simulink model "two_time_domains"  (R2025b)
settings: Solver=ode23tb  StartTime=0.0  StopTime=simlength  MaxStep=tc
undefined symbols (not defined in the file): dead_time_AFE, enable_pwm_phase_corrections, ki_align, kp_align, lim_down_align, lim_up_align, omega_base, tc, time_gain_afe_module_1, time_gain_afe_module_2, time_gain_inv_module_1, time_gain_inv_module_2, tPWM_AFE, tPWM_INV, ts_afe, ts_inv
settings Model: Creator=dbagn  LastModifiedBy=dbagn
settings SolverCC: NumberNewtonIterations=3.0  ZeroCrossControl=DisableAll  AlgebraicLoopSolver=TrustRegion  SolverResetMethod=Robust  AutoInsertRateTranBlk=on
settings DataIOCC: SaveOutput=off  SignalLogging=off  DSMLogging=off  SaveTime=off  ReturnWorkspaceOutputs=off
settings OptimizationCC: ReuseModelBlockBuffer=off
settings DebuggingCC: UnconnectedInputMsg=warning  UnconnectedOutputMsg=warning  UnconnectedLineMsg=warning
settings ModelReferenceCC: UpdateModelReferenceTargets=Force  EnableRefExpFcnMdlSchedulingChecks=on  ParallelModelReferenceMATLABWorkerInit=Copy Base Workspace
settings SFSimCC: CustomCodeUndefinedFunction=ThrowError  DefaultCustomCodeDeterministicFunctions=All
settings RTWCC: GPUComputeCapability=3.5  DLArmComputeVersion=19.05

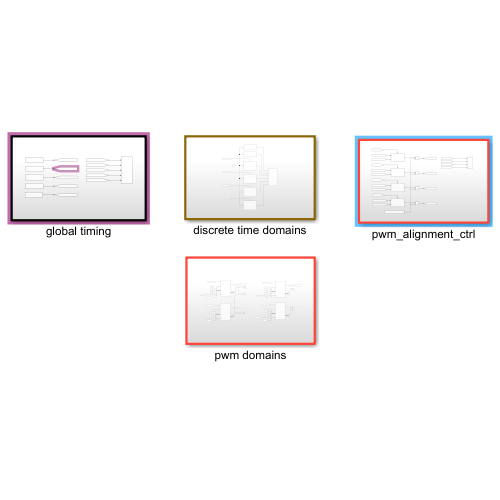
[thumbnail: Simulink's stored preview of the top-level diagram]
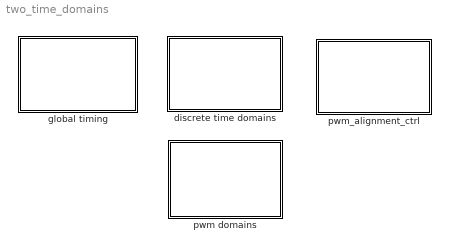
== system two_time_domains ==
  discrete time domains : Subsystem
  global timing : Subsystem
  pwm domains : Subsystem
  pwm_alignment_ctrl : Subsystem

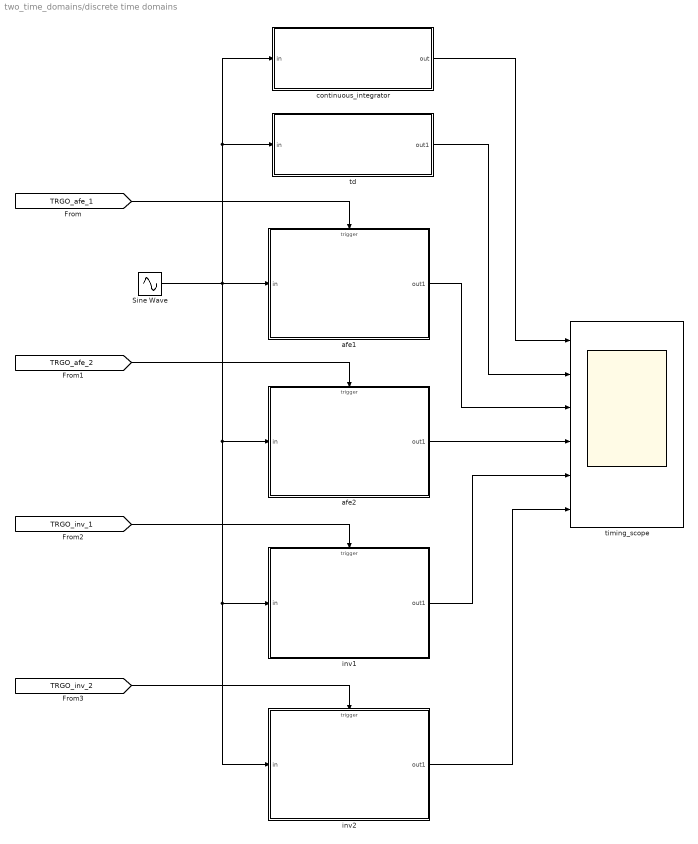
== system two_time_domains/discrete time domains ==
  Sine Wave : Sin  Frequency=omega_base  SampleTime=0
  afe1 : Subsystem
  afe2 : Subsystem
  continuous_integrator : Subsystem
  inv1 : Subsystem
  inv2 : Subsystem
  td : Subsystem
  timing_scope : Scope  NumInputPorts=6
      settings: SampleTime=tc  ActiveDisplayYMinimum=-0.89002047717580246  ActiveDisplayYMaximum=0.93911648822902838
  wires:
  [TRGO_afe_1] -> afe1/Trigger
  [TRGO_afe_2] -> afe2/Trigger
  Sine Wave/1 -> td/1(in), continuous_integrator/1(in), afe1/1(in), inv2/1(in), inv1/1(in), afe2/1(in)
  [TRGO_inv_2] -> inv2/Trigger
  [TRGO_inv_1] -> inv1/Trigger
  afe1/1(out1) -> timing_scope/3
  afe2/1(out1) -> timing_scope/4
  inv1/1(out1) -> timing_scope/5
  inv2/1(out1) -> timing_scope/6
  td/1(out1) -> timing_scope/2
  continuous_integrator/1(out) -> timing_scope/1

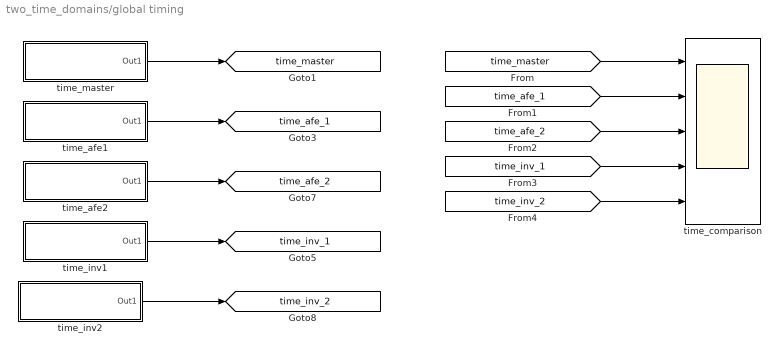
== system two_time_domains/global timing ==
  time_afe1 : Subsystem  mask{k=time_gain_afe_module_1}
      mask prompts: k "Time Gain"
      mask Display:
      | disp('time-gen');
      | port_label('output', 1, 'tout');
  time_afe2 : Subsystem  mask{k=time_gain_afe_module_2}
      mask prompts: k "Time Gain"
      mask Display:
      | disp('time-gen');
      | port_label('output', 1, 'tout');
  time_comparison : Scope  NumInputPorts=5
      settings: ActiveDisplayYMinimum=-0.0261093772199036  ActiveDisplayYMaximum=0.23498439497913245  DataLoggingVariableName=ScopeData6
  time_inv1 : Subsystem  mask{k=time_gain_inv_module_1}
      mask prompts: k "Time Gain"
      mask Display:
      | disp('time-gen');
      | port_label('output', 1, 'tout');
  time_inv2 : Subsystem  mask{k=time_gain_inv_module_2}
      mask prompts: k "Time Gain"
      mask Display:
      | disp('time-gen');
      | port_label('output', 1, 'tout');
  time_master : Subsystem  mask{k=1}
      mask prompts: k "Time Gain"
      mask Display:
      | disp('master');
      | port_label('output', 1, 'time');
  tag scope: time_afe_1=global, time_afe_2=global, time_inv_1=global, time_inv_2=global, time_master=global
  wires:
  time_afe1/1(Out1) -> [time_afe_1]
  time_afe2/1(Out1) -> [time_afe_2]
  time_master/1(Out1) -> [time_master]
  time_inv2/1(Out1) -> [time_inv_2]
  time_inv1/1(Out1) -> [time_inv_1]
  [time_master] -> time_comparison/1
  [time_afe_1] -> time_comparison/2
  [time_afe_2] -> time_comparison/3
  [time_inv_1] -> time_comparison/4
  [time_inv_2] -> time_comparison/5

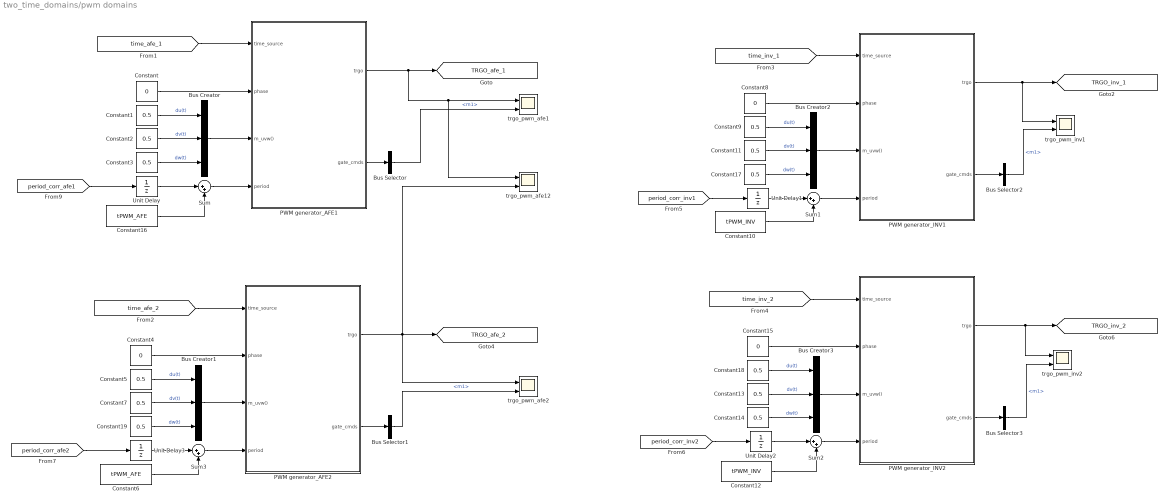
== system two_time_domains/pwm domains ==
  Bus Creator{,1..3} (4 alike) : BusCreator  Inputs=3
  Bus Selector{,1..3} (4 alike) : BusSelector  OutputSignals=m1
  Constant{,4,8,15} (4 alike) : Constant  Value=0
  Constant{1..3,5,7,9,11,13..14,17..19} (12 alike) : Constant  Value=0.5
  Constant10 : Constant  Value=tPWM_INV
  Constant12 : Constant  Value=tPWM_INV
  Constant16 : Constant  Value=tPWM_AFE
  Constant6 : Constant  Value=tPWM_AFE
  PWM generator_AFE1 : Subsystem  mask{m_up=0.98, m_low=0.02, dead_time=dead_time_AFE, pos_cmd_gate=15, neg_cmd_gate=-10, polarity=1, tc=tc}
      mask prompts: m_up "Max Input Modulation Value"; m_low "Min Input Modulation Value"; dead_time "Dead Time (s)"; pos_cmd_gate "Positive Gate Voltage (V)"; neg_cmd_gate "Negative Gate Voltage (V)"; polarity "Polarity (pu)"; tc "Sampling time"
  PWM generator_AFE2 : Subsystem  mask{m_up=0.98, m_low=0.02, dead_time=dead_time_AFE, pos_cmd_gate=15, neg_cmd_gate=-10, polarity=1, tc=tc}
      mask prompts: m_up "Max Input Modulation Value"; m_low "Min Input Modulation Value"; dead_time "Dead Time (s)"; pos_cmd_gate "Positive Gate Voltage (V)"; neg_cmd_gate "Negative Gate Voltage (V)"; polarity "Polarity (pu)"; tc "Sampling time"
  PWM generator_INV1 : Subsystem  mask{m_up=0.98, m_low=0.02, dead_time=dead_time_AFE, pos_cmd_gate=15, neg_cmd_gate=-10, polarity=1, tc=tc}
      mask prompts: m_up "Max Input Modulation Value"; m_low "Min Input Modulation Value"; dead_time "Dead Time (s)"; pos_cmd_gate "Positive Gate Voltage (V)"; neg_cmd_gate "Negative Gate Voltage (V)"; polarity "Polarity (pu)"; tc "Sampling time"
  PWM generator_INV2 : Subsystem  mask{m_up=0.98, m_low=0.02, dead_time=dead_time_AFE, pos_cmd_gate=15, neg_cmd_gate=-10, polarity=1, tc=tc}
      mask prompts: m_up "Max Input Modulation Value"; m_low "Min Input Modulation Value"; dead_time "Dead Time (s)"; pos_cmd_gate "Positive Gate Voltage (V)"; neg_cmd_gate "Negative Gate Voltage (V)"; polarity "Polarity (pu)"; tc "Sampling time"
  Sum{,1..3} (4 alike) : Sum  Inputs=|++
  Unit Delay{,1..3} (4 alike) : UnitDelay  InitialCondition=1  SampleTime=tc  HasFrameUpgradeWarning=on
  trgo_pwm_afe1 : Scope  NumInputPorts=2
      settings: ActiveDisplayYMinimum=-11.375  ActiveDisplayYMaximum=2.375
  trgo_pwm_afe12 : Scope  NumInputPorts=2
      settings: ActiveDisplayYMinimum=-1  ActiveDisplayYMaximum=1  DataLoggingVariableName=ScopeData5
  trgo_pwm_afe2 : Scope  NumInputPorts=2
      settings: ActiveDisplayYMinimum=-0.12499999999999997  ActiveDisplayYMaximum=1.125  DataLoggingVariableName=ScopeData2
  trgo_pwm_inv1 : Scope  NumInputPorts=2
      settings: ActiveDisplayYMinimum=-0.12499999999999997  ActiveDisplayYMaximum=1.125  DataLoggingVariableName=ScopeData3
  trgo_pwm_inv2 : Scope  NumInputPorts=2
      settings: ActiveDisplayYMinimum=-0.12499999999999997  ActiveDisplayYMaximum=1.125  DataLoggingVariableName=ScopeData4
  tag scope: TRGO_afe_1=global, TRGO_afe_2=global, TRGO_inv_1=global, TRGO_inv_2=global
  wires:
  Constant/1 -> PWM generator_AFE1/2(phase)
  Constant1/1 -> Bus Creator/1  "du(t)"
  [time_afe_1] -> PWM generator_AFE1/1(time_source)
  Bus Creator/1 -> PWM generator_AFE1/3(m_uvw())
  PWM generator_AFE1/1(trgo) -> trgo_pwm_afe12/1, trgo_pwm_afe1/1, [TRGO_afe_1]
  Constant2/1 -> Bus Creator/2  "dv(t)"
  Constant3/1 -> Bus Creator/3  "dw(t)"
  PWM generator_AFE1/2(gate_cmds) -> Bus Selector/1
  Bus Selector/1 -> trgo_pwm_afe1/2  "<m1>"
  Bus Selector1/1 -> trgo_pwm_afe2/2  "<m1>"
  PWM generator_AFE2/2(gate_cmds) -> Bus Selector1/1
  PWM generator_AFE2/1(trgo) -> trgo_pwm_afe12/2, [TRGO_afe_2], trgo_pwm_afe2/1
  [time_afe_2] -> PWM generator_AFE2/1(time_source)
  [time_inv_2] -> PWM generator_INV2/1(time_source)
  PWM generator_INV2/1(trgo) -> trgo_pwm_inv2/1, [TRGO_inv_2]
  PWM generator_INV2/2(gate_cmds) -> Bus Selector3/1
  Bus Selector3/1 -> trgo_pwm_inv2/2  "<m1>"
  Bus Selector2/1 -> trgo_pwm_inv1/2  "<m1>"
  PWM generator_INV1/2(gate_cmds) -> Bus Selector2/1
  PWM generator_INV1/1(trgo) -> [TRGO_inv_1], trgo_pwm_inv1/1
  [time_inv_1] -> PWM generator_INV1/1(time_source)
  Unit Delay/1 -> Sum/1
  [period_corr_afe1] -> Unit Delay/1
  Constant16/1 -> Sum/2
  Sum/1 -> PWM generator_AFE1/4(period)
  Constant10/1 -> Sum1/2
  [period_corr_inv1] -> Unit Delay1/1
  Constant9/1 -> Bus Creator2/1  "du(t)"
  Constant8/1 -> PWM generator_INV1/2(phase)
  Constant17/1 -> Bus Creator2/3  "dw(t)"
  Unit Delay1/1 -> Sum1/1
  Bus Creator2/1 -> PWM generator_INV1/3(m_uvw())
  Constant11/1 -> Bus Creator2/2  "dv(t)"
  Constant13/1 -> Bus Creator3/2  "dv(t)"
  Bus Creator3/1 -> PWM generator_INV2/3(m_uvw())
  Unit Delay2/1 -> Sum2/1
  Constant14/1 -> Bus Creator3/3  "dw(t)"
  Constant15/1 -> PWM generator_INV2/2(phase)
  Constant18/1 -> Bus Creator3/1  "du(t)"
  [period_corr_inv2] -> Unit Delay2/1
  Sum2/1 -> PWM generator_INV2/4(period)
  Constant12/1 -> Sum2/2
  Constant6/1 -> Sum3/2
  Sum3/1 -> PWM generator_AFE2/4(period)
  [period_corr_afe2] -> Unit Delay3/1
  Constant5/1 -> Bus Creator1/1  "du(t)"
  Constant4/1 -> PWM generator_AFE2/2(phase)
  Constant19/1 -> Bus Creator1/3  "dw(t)"
  Unit Delay3/1 -> Sum3/1
  Bus Creator1/1 -> PWM generator_AFE2/3(m_uvw())
  Constant7/1 -> Bus Creator1/2  "dv(t)"
  Sum1/1 -> PWM generator_INV1/4(period)

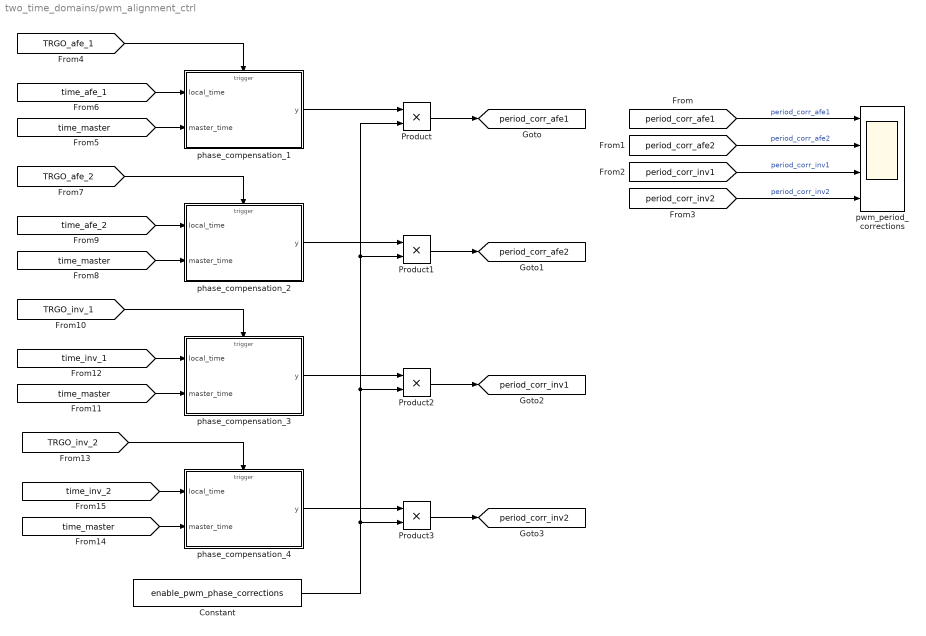
== system two_time_domains/pwm_alignment_ctrl ==
  Constant : Constant  Value=enable_pwm_phase_corrections
  Product{,1..3} (4 alike) : Product
  phase_compensation_1 : Subsystem
  phase_compensation_2 : Subsystem
  phase_compensation_3 : Subsystem
  phase_compensation_4 : Subsystem
  pwm_period_corrections : Scope  NumInputPorts=4
      settings: ActiveDisplayString=4  ActiveDisplayYMinimum=-6.4875940874999986E-5  ActiveDisplayYMaximum=7.2084378749999972E-6  DataLoggingVariableName=ScopeData7
  tag scope: period_corr_afe1=global, period_corr_afe2=global, period_corr_inv1=global, period_corr_inv2=global
  wires:
  Constant/1 -> Product1/2, Product/2, Product2/2, Product3/2
  Product/1 -> [period_corr_afe1]
  Product1/1 -> [period_corr_afe2]
  Product2/1 -> [period_corr_inv1]
  Product3/1 -> [period_corr_inv2]
  [period_corr_afe1] -> pwm_period_corrections/1  "period_corr_afe1"
  [period_corr_afe2] -> pwm_period_corrections/2  "period_corr_afe2"
  [period_corr_inv1] -> pwm_period_corrections/3  "period_corr_inv1"
  [period_corr_inv2] -> pwm_period_corrections/4  "period_corr_inv2"
  phase_compensation_1/1(y) -> Product/1
  [time_afe_1] -> phase_compensation_1/1(local_time)
  [time_master] -> phase_compensation_1/2(master_time)
  [time_master] -> phase_compensation_2/2(master_time)
  [time_afe_2] -> phase_compensation_2/1(local_time)
  phase_compensation_2/1(y) -> Product1/1
  [time_inv_1] -> phase_compensation_3/1(local_time)
  [time_master] -> phase_compensation_3/2(master_time)
  phase_compensation_3/1(y) -> Product2/1
  [time_master] -> phase_compensation_4/2(master_time)
  [time_inv_2] -> phase_compensation_4/1(local_time)
  phase_compensation_4/1(y) -> Product3/1
  [TRGO_afe_1] -> phase_compensation_1/Trigger
  [TRGO_inv_2] -> phase_compensation_4/Trigger
  [TRGO_inv_1] -> phase_compensation_3/Trigger
  [TRGO_afe_2] -> phase_compensation_2/Trigger

== system two_time_domains/discrete time domains/afe1 ==
  in : Inport
  Trigger : TriggerPort  VariantControl=(inherit)  PortDimensions=1
  LPF1_1 : Subsystem  mask{ts=ts_afe, omega=omega_base}
      mask Display:
      | disp('LPF1');
      | port_label('input', 1, 'u');
      | port_label('output', 1, 'y');
  out1 : Outport
  wires:
  in/1 -> LPF1_1/1(u)
  LPF1_1/1(y) -> out1/1

== system two_time_domains/discrete time domains/afe2 ==
  in : Inport
  Trigger : TriggerPort  VariantControl=(inherit)  PortDimensions=1
  LPF1_1 : Subsystem  mask{ts=ts_afe, omega=omega_base}
      mask Display:
      | disp('LPF1');
      | port_label('input', 1, 'u');
      | port_label('output', 1, 'y');
  out1 : Outport
  wires:
  LPF1_1/1(y) -> out1/1
  in/1 -> LPF1_1/1(u)

== system two_time_domains/discrete time domains/continuous_integrator ==
  in : Inport
  Transfer Fcn : TransferFcn  Denominator=[1/omega_base 1]
  out : Outport
  wires:
  in/1 -> Transfer Fcn/1
  Transfer Fcn/1 -> out/1

== system two_time_domains/discrete time domains/inv1 ==
  in : Inport
  Trigger : TriggerPort  VariantControl=(inherit)  PortDimensions=1
  LPF1_1 : Subsystem  mask{ts=ts_inv, omega=omega_base}
      mask Display:
      | disp('LPF1');
      | port_label('input', 1, 'u');
      | port_label('output', 1, 'y');
  out1 : Outport
  wires:
  in/1 -> LPF1_1/1(u)
  LPF1_1/1(y) -> out1/1

== system two_time_domains/discrete time domains/inv2 ==
  in : Inport
  Trigger : TriggerPort  VariantControl=(inherit)  PortDimensions=1
  LPF1_1 : Subsystem  mask{ts=ts_inv, omega=omega_base}
      mask Display:
      | disp('LPF1');
      | port_label('input', 1, 'u');
      | port_label('output', 1, 'y');
  out1 : Outport
  wires:
  LPF1_1/1(y) -> out1/1
  in/1 -> LPF1_1/1(u)

== system two_time_domains/discrete time domains/td ==
  in : Inport
  LPF1_1 : Subsystem  mask{ts=tc, omega=omega_base}
      mask Display:
      | disp('LPF1');
      | port_label('input', 1, 'u');
      | port_label('output', 1, 'y');
  out1 : Outport
  wires:
  LPF1_1/1(y) -> out1/1
  in/1 -> LPF1_1/1(u)

== system two_time_domains/global timing/time_afe1 ==
  Gain : Gain  Gain=k
  time_1 : Clock
  Out1 : Outport
  wires:
  time_1/1 -> Gain/1
  Gain/1 -> Out1/1

== system two_time_domains/global timing/time_afe2 ==
  Gain : Gain  Gain=k
  time_1 : Clock
  Out1 : Outport
  wires:
  Gain/1 -> Out1/1
  time_1/1 -> Gain/1

== system two_time_domains/global timing/time_inv1 ==
  Gain : Gain  Gain=k
  time_1 : Clock
  Out1 : Outport
  wires:
  time_1/1 -> Gain/1
  Gain/1 -> Out1/1

== system two_time_domains/global timing/time_inv2 ==
  Gain : Gain  Gain=k
  time_1 : Clock
  Out1 : Outport
  wires:
  Gain/1 -> Out1/1
  time_1/1 -> Gain/1

== system two_time_domains/global timing/time_master ==
  Gain : Gain  Gain=k
  time_1 : Clock
  Out1 : Outport
  wires:
  Gain/1 -> Out1/1
  time_1/1 -> Gain/1

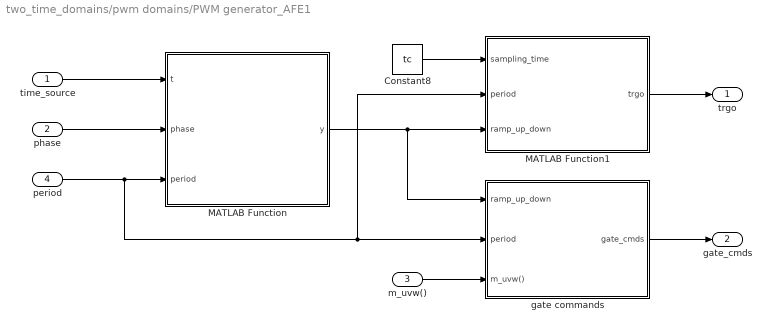
== system two_time_domains/pwm domains/PWM generator_AFE1 ==
  time_source : Inport
  phase : Inport  Port=2
  m_uvw() : Inport  Port=3
  period : Inport  Port=4
  Constant8 : Constant  Value=tc
  MATLAB Function : MATLAB Function  TreatAsAtomicUnit=on  SystemSampleTime=tc
  MATLAB Function1 : MATLAB Function  TreatAsAtomicUnit=on  SystemSampleTime=tc
  gate commands : Subsystem
  trgo : Outport
  gate_cmds : Outport  Port=2
  wires:
  phase/1 -> MATLAB Function/2(phase)
  MATLAB Function/1(y) -> gate commands/1(ramp_up_down), MATLAB Function1/3(ramp_up_down)
  MATLAB Function1/1(trgo) -> trgo/1
  Constant8/1 -> MATLAB Function1/1(sampling_time)
  period/1 -> MATLAB Function/3(period), MATLAB Function1/2(period), gate commands/2(period)
  m_uvw()/1 -> gate commands/3(m_uvw())
  gate commands/1(gate_cmds) -> gate_cmds/1
  time_source/1 -> MATLAB Function/1(t)

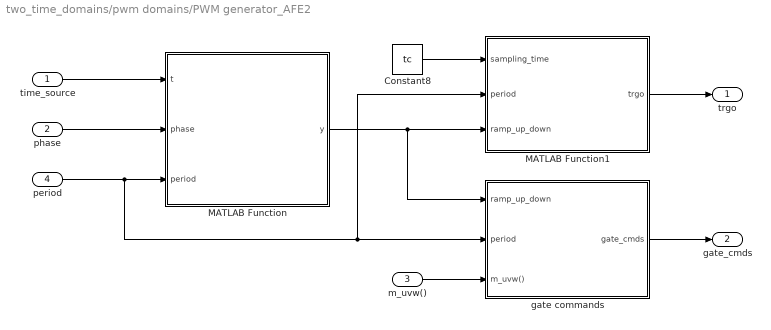
== system two_time_domains/pwm domains/PWM generator_AFE2 ==
  time_source : Inport
  phase : Inport  Port=2
  m_uvw() : Inport  Port=3
  period : Inport  Port=4
  Constant8 : Constant  Value=tc
  MATLAB Function : MATLAB Function  TreatAsAtomicUnit=on  SystemSampleTime=tc
  MATLAB Function1 : MATLAB Function  TreatAsAtomicUnit=on  SystemSampleTime=tc
  gate commands : Subsystem
  trgo : Outport
  gate_cmds : Outport  Port=2
  wires:
  time_source/1 -> MATLAB Function/1(t)
  gate commands/1(gate_cmds) -> gate_cmds/1
  m_uvw()/1 -> gate commands/3(m_uvw())
  period/1 -> gate commands/2(period), MATLAB Function1/2(period), MATLAB Function/3(period)
  Constant8/1 -> MATLAB Function1/1(sampling_time)
  MATLAB Function1/1(trgo) -> trgo/1
  MATLAB Function/1(y) -> MATLAB Function1/3(ramp_up_down), gate commands/1(ramp_up_down)
  phase/1 -> MATLAB Function/2(phase)

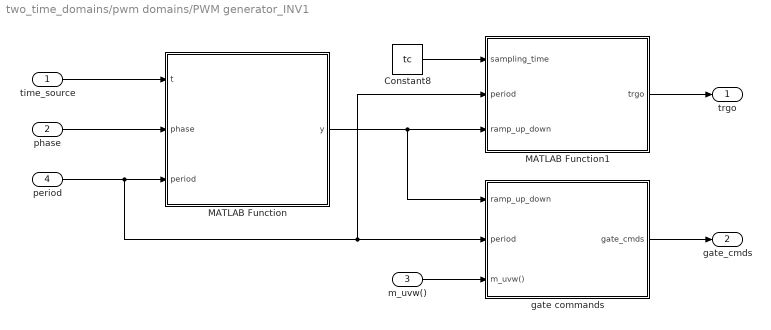
== system two_time_domains/pwm domains/PWM generator_INV1 ==
  time_source : Inport
  phase : Inport  Port=2
  m_uvw() : Inport  Port=3
  period : Inport  Port=4
  Constant8 : Constant  Value=tc
  MATLAB Function : MATLAB Function  TreatAsAtomicUnit=on  SystemSampleTime=tc
  MATLAB Function1 : MATLAB Function  TreatAsAtomicUnit=on  SystemSampleTime=tc
  gate commands : Subsystem
  trgo : Outport
  gate_cmds : Outport  Port=2
  wires:
  phase/1 -> MATLAB Function/2(phase)
  MATLAB Function/1(y) -> gate commands/1(ramp_up_down), MATLAB Function1/3(ramp_up_down)
  MATLAB Function1/1(trgo) -> trgo/1
  Constant8/1 -> MATLAB Function1/1(sampling_time)
  period/1 -> MATLAB Function/3(period), MATLAB Function1/2(period), gate commands/2(period)
  m_uvw()/1 -> gate commands/3(m_uvw())
  gate commands/1(gate_cmds) -> gate_cmds/1
  time_source/1 -> MATLAB Function/1(t)

== system two_time_domains/pwm domains/PWM generator_INV2 ==
  time_source : Inport
  phase : Inport  Port=2
  m_uvw() : Inport  Port=3
  period : Inport  Port=4
  Constant8 : Constant  Value=tc
  MATLAB Function : MATLAB Function  TreatAsAtomicUnit=on  SystemSampleTime=tc
  MATLAB Function1 : MATLAB Function  TreatAsAtomicUnit=on  SystemSampleTime=tc
  gate commands : Subsystem
  trgo : Outport
  gate_cmds : Outport  Port=2
  wires:
  time_source/1 -> MATLAB Function/1(t)
  gate commands/1(gate_cmds) -> gate_cmds/1
  m_uvw()/1 -> gate commands/3(m_uvw())
  period/1 -> gate commands/2(period), MATLAB Function1/2(period), MATLAB Function/3(period)
  Constant8/1 -> MATLAB Function1/1(sampling_time)
  MATLAB Function1/1(trgo) -> trgo/1
  MATLAB Function/1(y) -> MATLAB Function1/3(ramp_up_down), gate commands/1(ramp_up_down)
  phase/1 -> MATLAB Function/2(phase)

== system two_time_domains/pwm_alignment_ctrl/phase_compensation_1 ==
  local_time : Inport
  master_time : Inport  Port=2
  Trigger : TriggerPort  VariantControl=(inherit)  PortDimensions=1
  Gain1 : Gain  Gain=tPWM_AFE
  alignment_pictrl : Subsystem
  y : Outport
  wires:
  local_time/1 -> alignment_pictrl/1(local_time)
  master_time/1 -> alignment_pictrl/2(master_time)
  alignment_pictrl/1(dp) -> Gain1/1
  Gain1/1 -> y/1

== system two_time_domains/pwm_alignment_ctrl/phase_compensation_2 ==
  local_time : Inport
  master_time : Inport  Port=2
  Trigger : TriggerPort  VariantControl=(inherit)  PortDimensions=1
  Gain1 : Gain  Gain=tPWM_AFE
  alignment_pictrl : Subsystem
  y : Outport
  wires:
  alignment_pictrl/1(dp) -> Gain1/1
  master_time/1 -> alignment_pictrl/2(master_time)
  local_time/1 -> alignment_pictrl/1(local_time)
  Gain1/1 -> y/1

== system two_time_domains/pwm_alignment_ctrl/phase_compensation_3 ==
  local_time : Inport
  master_time : Inport  Port=2
  Trigger : TriggerPort  VariantControl=(inherit)  PortDimensions=1
  Gain1 : Gain  Gain=tPWM_INV
  alignment_pictrl : Subsystem
  y : Outport
  wires:
  local_time/1 -> alignment_pictrl/1(local_time)
  master_time/1 -> alignment_pictrl/2(master_time)
  alignment_pictrl/1(dp) -> Gain1/1
  Gain1/1 -> y/1

== system two_time_domains/pwm_alignment_ctrl/phase_compensation_4 ==
  local_time : Inport
  master_time : Inport  Port=2
  Trigger : TriggerPort  VariantControl=(inherit)  PortDimensions=1
  Gain1 : Gain  Gain=tPWM_INV
  alignment_pictrl : Subsystem
  y : Outport
  wires:
  alignment_pictrl/1(dp) -> Gain1/1
  master_time/1 -> alignment_pictrl/2(master_time)
  local_time/1 -> alignment_pictrl/1(local_time)
  Gain1/1 -> y/1

== system two_time_domains/discrete time domains/afe1/LPF1_1 ==
  u : Inport
  Gain : Gain  Gain=1-exp(-omega*ts)
  Gain1 : Gain  Gain=exp(-omega*ts)
  Sum : Sum  Inputs=|++
  Unit Delay : UnitDelay  SampleTime=-1  HasFrameUpgradeWarning=on
  y : Outport
  wires:
  Gain1/1 -> Sum/2
  Unit Delay/1 -> y/1, Gain1/1
  Gain/1 -> Sum/1
  Sum/1 -> Unit Delay/1
  u/1 -> Gain/1

== system two_time_domains/discrete time domains/afe2/LPF1_1 ==
  u : Inport
  Gain : Gain  Gain=1-exp(-omega*ts)
  Gain1 : Gain  Gain=exp(-omega*ts)
  Sum : Sum  Inputs=|++
  Unit Delay : UnitDelay  SampleTime=-1  HasFrameUpgradeWarning=on
  y : Outport
  wires:
  u/1 -> Gain/1
  Sum/1 -> Unit Delay/1
  Gain/1 -> Sum/1
  Unit Delay/1 -> Gain1/1, y/1
  Gain1/1 -> Sum/2

== system two_time_domains/discrete time domains/inv1/LPF1_1 ==
  u : Inport
  Gain : Gain  Gain=1-exp(-omega*ts)
  Gain1 : Gain  Gain=exp(-omega*ts)
  Sum : Sum  Inputs=|++
  Unit Delay : UnitDelay  SampleTime=-1  HasFrameUpgradeWarning=on
  y : Outport
  wires:
  Gain1/1 -> Sum/2
  Unit Delay/1 -> y/1, Gain1/1
  Gain/1 -> Sum/1
  Sum/1 -> Unit Delay/1
  u/1 -> Gain/1

== system two_time_domains/discrete time domains/inv2/LPF1_1 ==
  u : Inport
  Gain : Gain  Gain=1-exp(-omega*ts)
  Gain1 : Gain  Gain=exp(-omega*ts)
  Sum : Sum  Inputs=|++
  Unit Delay : UnitDelay  SampleTime=-1  HasFrameUpgradeWarning=on
  y : Outport
  wires:
  u/1 -> Gain/1
  Sum/1 -> Unit Delay/1
  Gain/1 -> Sum/1
  Unit Delay/1 -> Gain1/1, y/1
  Gain1/1 -> Sum/2

== system two_time_domains/discrete time domains/td/LPF1_1 ==
  u : Inport
  Gain : Gain  Gain=1-exp(-omega*ts)
  Gain1 : Gain  Gain=exp(-omega*ts)
  Sum : Sum  Inputs=|++
  Unit Delay : UnitDelay  SampleTime=-1  HasFrameUpgradeWarning=on
  y : Outport
  wires:
  u/1 -> Gain/1
  Sum/1 -> Unit Delay/1
  Gain/1 -> Sum/1
  Unit Delay/1 -> Gain1/1, y/1
  Gain1/1 -> Sum/2

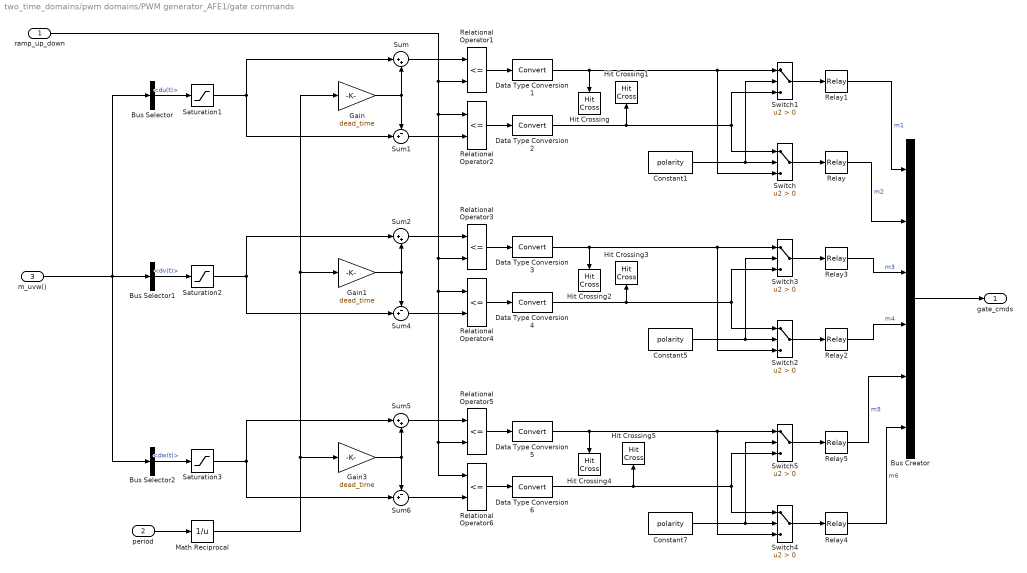
== system two_time_domains/pwm domains/PWM generator_AFE1/gate commands ==
  ramp_up_down : Inport
  period : Inport  Port=2
  m_uvw() : Inport  Port=3
  Bus Creator : BusCreator  Inputs=6
  Bus Selector : BusSelector  OutputSignals=du(t)
  Bus Selector1 : BusSelector  OutputSignals=dv(t)
  Bus Selector2 : BusSelector  OutputSignals=dw(t)
  Constant1 : Constant  Value=polarity
  Constant5 : Constant  Value=polarity
  Constant7 : Constant  Value=polarity
  Data Type Conversion{1..6} (6 alike) : DataTypeConversion
  Gain : Gain  Gain=dead_time
  Gain1 : Gain  Gain=dead_time
  Gain3 : Gain  Gain=dead_time
  Hit Crossing{,1..5} (6 alike) : HitCross  ShowOutputPort=off
  Math Reciprocal : Math  Operator=reciprocal  SignedPower=on
  Relational Operator{1..6} (6 alike) : RelationalOperator  Operator=<=  InputSameDT=off
  Relay{,1..5} (6 alike) : Relay  OnOutputValue=pos_cmd_gate  OffOutputValue=neg_cmd_gate
  Saturation1 : Saturate  UpperLimit=m_up  LowerLimit=m_low
  Saturation2 : Saturate  UpperLimit=m_up  LowerLimit=m_low
  Saturation3 : Saturate  UpperLimit=m_up  LowerLimit=m_low
  Sum : Sum  Inputs=|++  SaturateOnIntegerOverflow=on
  Sum1 : Sum  Inputs=-+|  SaturateOnIntegerOverflow=on
  Sum2 : Sum  Inputs=|++  SaturateOnIntegerOverflow=on
  Sum4 : Sum  Inputs=-+|  SaturateOnIntegerOverflow=on
  Sum5 : Sum  Inputs=|++  SaturateOnIntegerOverflow=on
  Sum6 : Sum  Inputs=-+|  SaturateOnIntegerOverflow=on
  Switch{,1..5} (6 alike) : Switch  Criteria=u2 > Threshold  SaturateOnIntegerOverflow=off  InputSameDT=off
  gate_cmds : Outport
  wires:
  Data Type Conversion6/1 -> Switch4/1, Switch5/3, Hit Crossing5/1
  Constant1/1 -> Switch1/2, Switch/2
  Data Type Conversion1/1 -> Switch/3, Switch1/1, Hit Crossing/1
  Gain1/1 -> Sum4/1, Sum2/2
  m_uvw()/1 -> Bus Selector/1, Bus Selector2/1, Bus Selector1/1
  Relay4/1 -> Bus Creator/6  "m6"
  Gain3/1 -> Sum5/2, Sum6/1
  Saturation1/1 -> Sum1/2, Sum/1
  Data Type Conversion3/1 -> Switch2/3, Switch3/1, Hit Crossing2/1
  Data Type Conversion2/1 -> Switch/1, Switch1/3, Hit Crossing1/1
  Relational Operator1/1 -> Data Type Conversion1/1
  Bus Creator/1 -> gate_cmds/1
  Data Type Conversion5/1 -> Switch4/3, Switch5/1, Hit Crossing4/1
  Sum1/1 -> Relational Operator2/2
  Constant5/1 -> Switch2/2, Switch3/2
  Switch/1 -> Relay/1
  Sum/1 -> Relational Operator1/1
  Relational Operator6/1 -> Data Type Conversion6/1
  Relay2/1 -> Bus Creator/4  "m4"
  Saturation3/1 -> Sum5/1, Sum6/2
  Constant7/1 -> Switch5/2, Switch4/2
  Sum5/1 -> Relational Operator5/1
  Bus Selector/1 -> Saturation1/1  "<du(t)>"
  Data Type Conversion4/1 -> Switch2/1, Switch3/3, Hit Crossing3/1
  ramp_up_down/1 -> Relational Operator3/2, Relational Operator6/1, Relational Operator5/2, Relational Operator4/1, Relational Operator2/1, Relational Operator1/2
  Switch4/1 -> Relay4/1
  Relational Operator5/1 -> Data Type Conversion5/1
  Switch5/1 -> Relay5/1
  Saturation2/1 -> Sum4/2, Sum2/1
  Relational Operator3/1 -> Data Type Conversion3/1
  Sum2/1 -> Relational Operator3/1
  Switch1/1 -> Relay1/1
  Relay3/1 -> Bus Creator/3  "m3"
  Relational Operator2/1 -> Data Type Conversion2/1
  Bus Selector1/1 -> Saturation2/1  "<dv(t)>"
  Switch3/1 -> Relay3/1
  Sum4/1 -> Relational Operator4/2
  Relay/1 -> Bus Creator/2  "m2"
  Relational Operator4/1 -> Data Type Conversion4/1
  Bus Selector2/1 -> Saturation3/1  "<dw(t)>"
  Relay1/1 -> Bus Creator/1  "m1"
  Sum6/1 -> Relational Operator6/2
  Gain/1 -> Sum1/1, Sum/2
  Relay5/1 -> Bus Creator/5  "m5"
  Switch2/1 -> Relay2/1
  period/1 -> Math Reciprocal/1
  Math Reciprocal/1 -> Gain3/1, Gain1/1, Gain/1

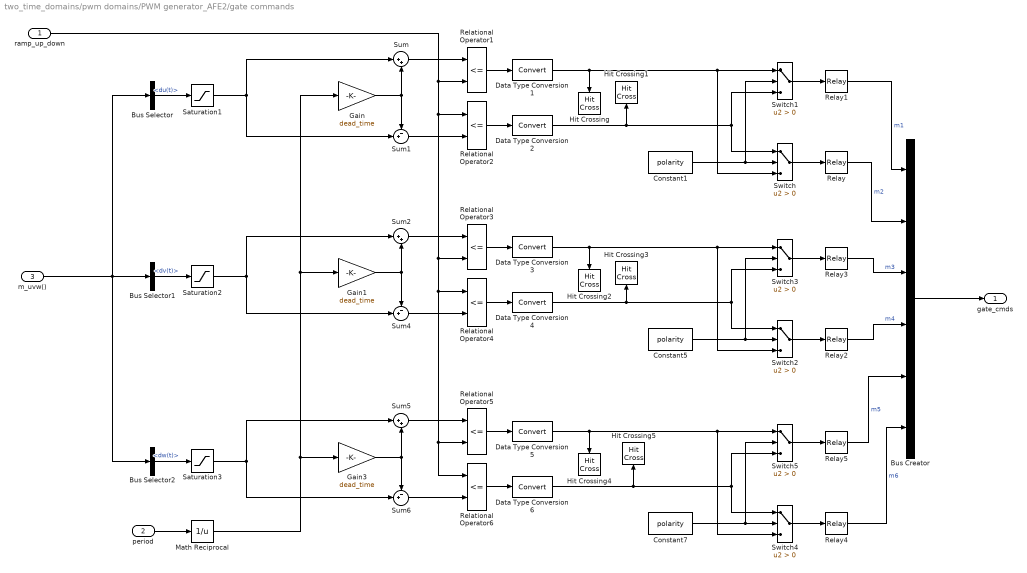
== system two_time_domains/pwm domains/PWM generator_AFE2/gate commands ==
  ramp_up_down : Inport
  period : Inport  Port=2
  m_uvw() : Inport  Port=3
  Bus Creator : BusCreator  Inputs=6
  Bus Selector : BusSelector  OutputSignals=du(t)
  Bus Selector1 : BusSelector  OutputSignals=dv(t)
  Bus Selector2 : BusSelector  OutputSignals=dw(t)
  Constant1 : Constant  Value=polarity
  Constant5 : Constant  Value=polarity
  Constant7 : Constant  Value=polarity
  Data Type Conversion{1..6} (6 alike) : DataTypeConversion
  Gain : Gain  Gain=dead_time
  Gain1 : Gain  Gain=dead_time
  Gain3 : Gain  Gain=dead_time
  Hit Crossing{,1..5} (6 alike) : HitCross  ShowOutputPort=off
  Math Reciprocal : Math  Operator=reciprocal  SignedPower=on
  Relational Operator{1..6} (6 alike) : RelationalOperator  Operator=<=  InputSameDT=off
  Relay{,1..5} (6 alike) : Relay  OnOutputValue=pos_cmd_gate  OffOutputValue=neg_cmd_gate
  Saturation1 : Saturate  UpperLimit=m_up  LowerLimit=m_low
  Saturation2 : Saturate  UpperLimit=m_up  LowerLimit=m_low
  Saturation3 : Saturate  UpperLimit=m_up  LowerLimit=m_low
  Sum : Sum  Inputs=|++  SaturateOnIntegerOverflow=on
  Sum1 : Sum  Inputs=-+|  SaturateOnIntegerOverflow=on
  Sum2 : Sum  Inputs=|++  SaturateOnIntegerOverflow=on
  Sum4 : Sum  Inputs=-+|  SaturateOnIntegerOverflow=on
  Sum5 : Sum  Inputs=|++  SaturateOnIntegerOverflow=on
  Sum6 : Sum  Inputs=-+|  SaturateOnIntegerOverflow=on
  Switch{,1..5} (6 alike) : Switch  Criteria=u2 > Threshold  SaturateOnIntegerOverflow=off  InputSameDT=off
  gate_cmds : Outport
  wires:
  Math Reciprocal/1 -> Gain/1, Gain1/1, Gain3/1
  period/1 -> Math Reciprocal/1
  Switch2/1 -> Relay2/1
  Relay5/1 -> Bus Creator/5  "m5"
  Gain/1 -> Sum/2, Sum1/1
  Sum6/1 -> Relational Operator6/2
  Relay1/1 -> Bus Creator/1  "m1"
  Bus Selector2/1 -> Saturation3/1  "<dw(t)>"
  Relational Operator4/1 -> Data Type Conversion4/1
  Relay/1 -> Bus Creator/2  "m2"
  Sum4/1 -> Relational Operator4/2
  Switch3/1 -> Relay3/1
  Bus Selector1/1 -> Saturation2/1  "<dv(t)>"
  Relational Operator2/1 -> Data Type Conversion2/1
  Relay3/1 -> Bus Creator/3  "m3"
  Switch1/1 -> Relay1/1
  Sum2/1 -> Relational Operator3/1
  Relational Operator3/1 -> Data Type Conversion3/1
  Saturation2/1 -> Sum2/1, Sum4/2
  Switch5/1 -> Relay5/1
  Relational Operator5/1 -> Data Type Conversion5/1
  Switch4/1 -> Relay4/1
  ramp_up_down/1 -> Relational Operator1/2, Relational Operator2/1, Relational Operator4/1, Relational Operator5/2, Relational Operator6/1, Relational Operator3/2
  Data Type Conversion4/1 -> Hit Crossing3/1, Switch3/3, Switch2/1
  Bus Selector/1 -> Saturation1/1  "<du(t)>"
  Sum5/1 -> Relational Operator5/1
  Constant7/1 -> Switch4/2, Switch5/2
  Saturation3/1 -> Sum6/2, Sum5/1
  Relay2/1 -> Bus Creator/4  "m4"
  Relational Operator6/1 -> Data Type Conversion6/1
  Sum/1 -> Relational Operator1/1
  Switch/1 -> Relay/1
  Constant5/1 -> Switch3/2, Switch2/2
  Sum1/1 -> Relational Operator2/2
  Data Type Conversion5/1 -> Hit Crossing4/1, Switch5/1, Switch4/3
  Bus Creator/1 -> gate_cmds/1
  Relational Operator1/1 -> Data Type Conversion1/1
  Data Type Conversion2/1 -> Hit Crossing1/1, Switch1/3, Switch/1
  Data Type Conversion3/1 -> Hit Crossing2/1, Switch3/1, Switch2/3
  Saturation1/1 -> Sum/1, Sum1/2
  Gain3/1 -> Sum6/1, Sum5/2
  Relay4/1 -> Bus Creator/6  "m6"
  m_uvw()/1 -> Bus Selector1/1, Bus Selector2/1, Bus Selector/1
  Gain1/1 -> Sum2/2, Sum4/1
  Data Type Conversion1/1 -> Hit Crossing/1, Switch1/1, Switch/3
  Constant1/1 -> Switch/2, Switch1/2
  Data Type Conversion6/1 -> Hit Crossing5/1, Switch5/3, Switch4/1

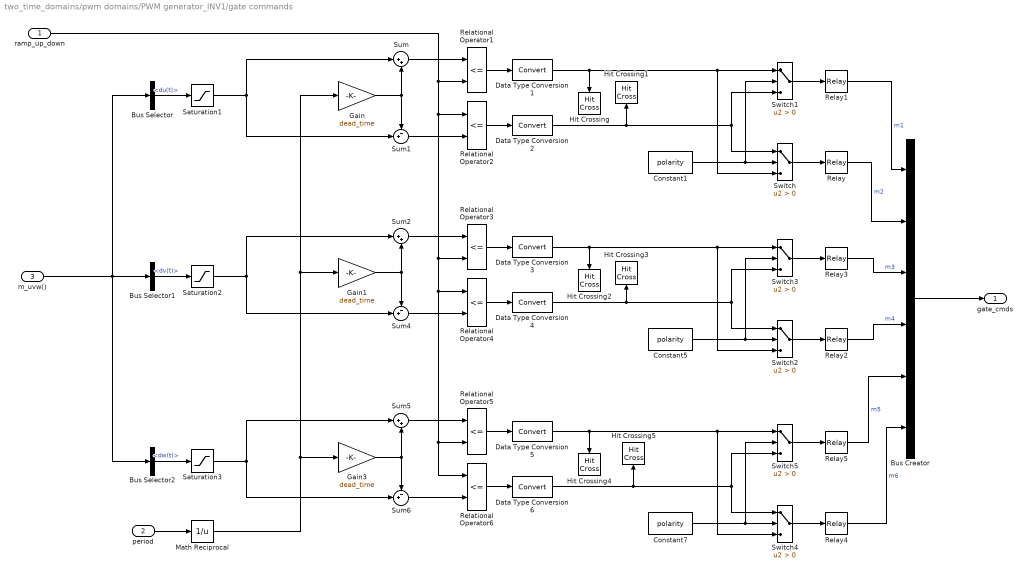
== system two_time_domains/pwm domains/PWM generator_INV1/gate commands ==
  ramp_up_down : Inport
  period : Inport  Port=2
  m_uvw() : Inport  Port=3
  Bus Creator : BusCreator  Inputs=6
  Bus Selector : BusSelector  OutputSignals=du(t)
  Bus Selector1 : BusSelector  OutputSignals=dv(t)
  Bus Selector2 : BusSelector  OutputSignals=dw(t)
  Constant1 : Constant  Value=polarity
  Constant5 : Constant  Value=polarity
  Constant7 : Constant  Value=polarity
  Data Type Conversion{1..6} (6 alike) : DataTypeConversion
  Gain : Gain  Gain=dead_time
  Gain1 : Gain  Gain=dead_time
  Gain3 : Gain  Gain=dead_time
  Hit Crossing{,1..5} (6 alike) : HitCross  ShowOutputPort=off
  Math Reciprocal : Math  Operator=reciprocal  SignedPower=on
  Relational Operator{1..6} (6 alike) : RelationalOperator  Operator=<=  InputSameDT=off
  Relay{,1..5} (6 alike) : Relay  OnOutputValue=pos_cmd_gate  OffOutputValue=neg_cmd_gate
  Saturation1 : Saturate  UpperLimit=m_up  LowerLimit=m_low
  Saturation2 : Saturate  UpperLimit=m_up  LowerLimit=m_low
  Saturation3 : Saturate  UpperLimit=m_up  LowerLimit=m_low
  Sum : Sum  Inputs=|++  SaturateOnIntegerOverflow=on
  Sum1 : Sum  Inputs=-+|  SaturateOnIntegerOverflow=on
  Sum2 : Sum  Inputs=|++  SaturateOnIntegerOverflow=on
  Sum4 : Sum  Inputs=-+|  SaturateOnIntegerOverflow=on
  Sum5 : Sum  Inputs=|++  SaturateOnIntegerOverflow=on
  Sum6 : Sum  Inputs=-+|  SaturateOnIntegerOverflow=on
  Switch{,1..5} (6 alike) : Switch  Criteria=u2 > Threshold  SaturateOnIntegerOverflow=off  InputSameDT=off
  gate_cmds : Outport
  wires:
  Data Type Conversion6/1 -> Switch4/1, Switch5/3, Hit Crossing5/1
  Constant1/1 -> Switch1/2, Switch/2
  Data Type Conversion1/1 -> Switch/3, Switch1/1, Hit Crossing/1
  Gain1/1 -> Sum4/1, Sum2/2
  m_uvw()/1 -> Bus Selector/1, Bus Selector2/1, Bus Selector1/1
  Relay4/1 -> Bus Creator/6  "m6"
  Gain3/1 -> Sum5/2, Sum6/1
  Saturation1/1 -> Sum1/2, Sum/1
  Data Type Conversion3/1 -> Switch2/3, Switch3/1, Hit Crossing2/1
  Data Type Conversion2/1 -> Switch/1, Switch1/3, Hit Crossing1/1
  Relational Operator1/1 -> Data Type Conversion1/1
  Bus Creator/1 -> gate_cmds/1
  Data Type Conversion5/1 -> Switch4/3, Switch5/1, Hit Crossing4/1
  Sum1/1 -> Relational Operator2/2
  Constant5/1 -> Switch2/2, Switch3/2
  Switch/1 -> Relay/1
  Sum/1 -> Relational Operator1/1
  Relational Operator6/1 -> Data Type Conversion6/1
  Relay2/1 -> Bus Creator/4  "m4"
  Saturation3/1 -> Sum5/1, Sum6/2
  Constant7/1 -> Switch5/2, Switch4/2
  Sum5/1 -> Relational Operator5/1
  Bus Selector/1 -> Saturation1/1  "<du(t)>"
  Data Type Conversion4/1 -> Switch2/1, Switch3/3, Hit Crossing3/1
  ramp_up_down/1 -> Relational Operator3/2, Relational Operator6/1, Relational Operator5/2, Relational Operator4/1, Relational Operator2/1, Relational Operator1/2
  Switch4/1 -> Relay4/1
  Relational Operator5/1 -> Data Type Conversion5/1
  Switch5/1 -> Relay5/1
  Saturation2/1 -> Sum4/2, Sum2/1
  Relational Operator3/1 -> Data Type Conversion3/1
  Sum2/1 -> Relational Operator3/1
  Switch1/1 -> Relay1/1
  Relay3/1 -> Bus Creator/3  "m3"
  Relational Operator2/1 -> Data Type Conversion2/1
  Bus Selector1/1 -> Saturation2/1  "<dv(t)>"
  Switch3/1 -> Relay3/1
  Sum4/1 -> Relational Operator4/2
  Relay/1 -> Bus Creator/2  "m2"
  Relational Operator4/1 -> Data Type Conversion4/1
  Bus Selector2/1 -> Saturation3/1  "<dw(t)>"
  Relay1/1 -> Bus Creator/1  "m1"
  Sum6/1 -> Relational Operator6/2
  Gain/1 -> Sum1/1, Sum/2
  Relay5/1 -> Bus Creator/5  "m5"
  Switch2/1 -> Relay2/1
  period/1 -> Math Reciprocal/1
  Math Reciprocal/1 -> Gain3/1, Gain1/1, Gain/1

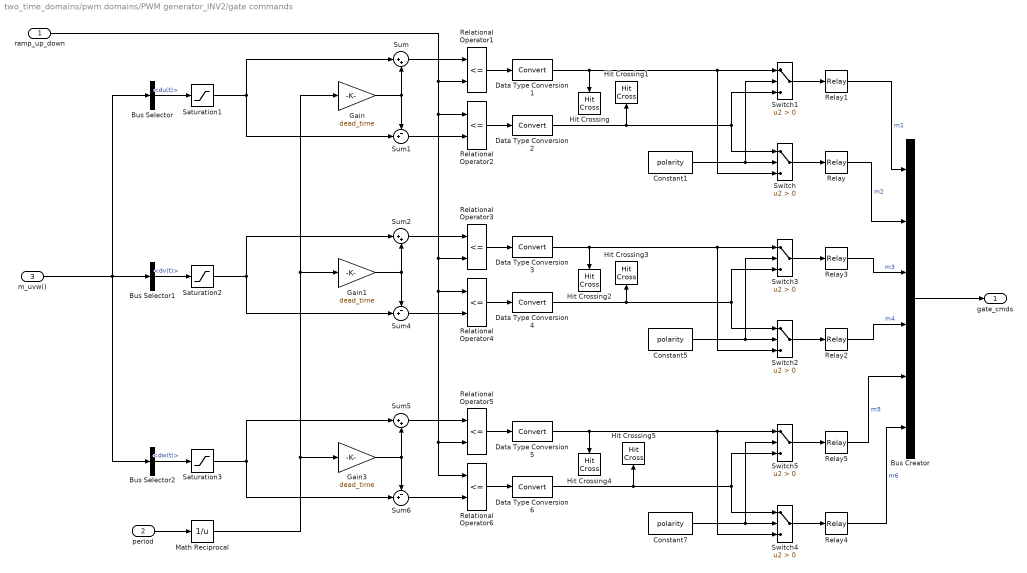
== system two_time_domains/pwm domains/PWM generator_INV2/gate commands ==
  ramp_up_down : Inport
  period : Inport  Port=2
  m_uvw() : Inport  Port=3
  Bus Creator : BusCreator  Inputs=6
  Bus Selector : BusSelector  OutputSignals=du(t)
  Bus Selector1 : BusSelector  OutputSignals=dv(t)
  Bus Selector2 : BusSelector  OutputSignals=dw(t)
  Constant1 : Constant  Value=polarity
  Constant5 : Constant  Value=polarity
  Constant7 : Constant  Value=polarity
  Data Type Conversion{1..6} (6 alike) : DataTypeConversion
  Gain : Gain  Gain=dead_time
  Gain1 : Gain  Gain=dead_time
  Gain3 : Gain  Gain=dead_time
  Hit Crossing{,1..5} (6 alike) : HitCross  ShowOutputPort=off
  Math Reciprocal : Math  Operator=reciprocal  SignedPower=on
  Relational Operator{1..6} (6 alike) : RelationalOperator  Operator=<=  InputSameDT=off
  Relay{,1..5} (6 alike) : Relay  OnOutputValue=pos_cmd_gate  OffOutputValue=neg_cmd_gate
  Saturation1 : Saturate  UpperLimit=m_up  LowerLimit=m_low
  Saturation2 : Saturate  UpperLimit=m_up  LowerLimit=m_low
  Saturation3 : Saturate  UpperLimit=m_up  LowerLimit=m_low
  Sum : Sum  Inputs=|++  SaturateOnIntegerOverflow=on
  Sum1 : Sum  Inputs=-+|  SaturateOnIntegerOverflow=on
  Sum2 : Sum  Inputs=|++  SaturateOnIntegerOverflow=on
  Sum4 : Sum  Inputs=-+|  SaturateOnIntegerOverflow=on
  Sum5 : Sum  Inputs=|++  SaturateOnIntegerOverflow=on
  Sum6 : Sum  Inputs=-+|  SaturateOnIntegerOverflow=on
  Switch{,1..5} (6 alike) : Switch  Criteria=u2 > Threshold  SaturateOnIntegerOverflow=off  InputSameDT=off
  gate_cmds : Outport
  wires:
  Math Reciprocal/1 -> Gain/1, Gain1/1, Gain3/1
  period/1 -> Math Reciprocal/1
  Switch2/1 -> Relay2/1
  Relay5/1 -> Bus Creator/5  "m5"
  Gain/1 -> Sum/2, Sum1/1
  Sum6/1 -> Relational Operator6/2
  Relay1/1 -> Bus Creator/1  "m1"
  Bus Selector2/1 -> Saturation3/1  "<dw(t)>"
  Relational Operator4/1 -> Data Type Conversion4/1
  Relay/1 -> Bus Creator/2  "m2"
  Sum4/1 -> Relational Operator4/2
  Switch3/1 -> Relay3/1
  Bus Selector1/1 -> Saturation2/1  "<dv(t)>"
  Relational Operator2/1 -> Data Type Conversion2/1
  Relay3/1 -> Bus Creator/3  "m3"
  Switch1/1 -> Relay1/1
  Sum2/1 -> Relational Operator3/1
  Relational Operator3/1 -> Data Type Conversion3/1
  Saturation2/1 -> Sum2/1, Sum4/2
  Switch5/1 -> Relay5/1
  Relational Operator5/1 -> Data Type Conversion5/1
  Switch4/1 -> Relay4/1
  ramp_up_down/1 -> Relational Operator1/2, Relational Operator2/1, Relational Operator4/1, Relational Operator5/2, Relational Operator6/1, Relational Operator3/2
  Data Type Conversion4/1 -> Hit Crossing3/1, Switch3/3, Switch2/1
  Bus Selector/1 -> Saturation1/1  "<du(t)>"
  Sum5/1 -> Relational Operator5/1
  Constant7/1 -> Switch4/2, Switch5/2
  Saturation3/1 -> Sum6/2, Sum5/1
  Relay2/1 -> Bus Creator/4  "m4"
  Relational Operator6/1 -> Data Type Conversion6/1
  Sum/1 -> Relational Operator1/1
  Switch/1 -> Relay/1
  Constant5/1 -> Switch3/2, Switch2/2
  Sum1/1 -> Relational Operator2/2
  Data Type Conversion5/1 -> Hit Crossing4/1, Switch5/1, Switch4/3
  Bus Creator/1 -> gate_cmds/1
  Relational Operator1/1 -> Data Type Conversion1/1
  Data Type Conversion2/1 -> Hit Crossing1/1, Switch1/3, Switch/1
  Data Type Conversion3/1 -> Hit Crossing2/1, Switch3/1, Switch2/3
  Saturation1/1 -> Sum/1, Sum1/2
  Gain3/1 -> Sum6/1, Sum5/2
  Relay4/1 -> Bus Creator/6  "m6"
  m_uvw()/1 -> Bus Selector1/1, Bus Selector2/1, Bus Selector/1
  Gain1/1 -> Sum2/2, Sum4/1
  Data Type Conversion1/1 -> Hit Crossing/1, Switch1/1, Switch/3
  Constant1/1 -> Switch/2, Switch1/2
  Data Type Conversion6/1 -> Hit Crossing5/1, Switch5/3, Switch4/1

== system two_time_domains/pwm_alignment_ctrl/phase_compensation_1/alignment_pictrl ==
  local_time : Inport
  master_time : Inport  Port=2
  Constant : Constant  Value=0
  Sum : Sum  Inputs=|+-
  pi : Subsystem  mask{kp=kp_align, ki=ki_align, lim_up=lim_up_align, lim_down=lim_down_align}
      mask prompts: ki "ki*ts"
      mask Display:
      | disp('pi()');
      | port_label('input', 1, 'u_ref');
      | port_label('input', 2, 'u');
      | port_label('output', 1, 'y');
  dp : Outport
  wires:
  master_time/1 -> Sum/1
  Constant/1 -> pi/1(u_ref)
  local_time/1 -> Sum/2
  Sum/1 -> pi/2(u)
  pi/1(y) -> dp/1

== system two_time_domains/pwm_alignment_ctrl/phase_compensation_2/alignment_pictrl ==
  local_time : Inport
  master_time : Inport  Port=2
  Constant : Constant  Value=0
  Sum : Sum  Inputs=|+-
  pi : Subsystem  mask{kp=kp_align, ki=ki_align, lim_up=lim_up_align, lim_down=lim_down_align}
      mask prompts: ki "ki*ts"
      mask Display:
      | disp('pi()');
      | port_label('input', 1, 'u_ref');
      | port_label('input', 2, 'u');
      | port_label('output', 1, 'y');
  dp : Outport
  wires:
  master_time/1 -> Sum/1
  local_time/1 -> Sum/2
  Constant/1 -> pi/1(u_ref)
  Sum/1 -> pi/2(u)
  pi/1(y) -> dp/1

== system two_time_domains/pwm_alignment_ctrl/phase_compensation_3/alignment_pictrl ==
  local_time : Inport
  master_time : Inport  Port=2
  Constant : Constant  Value=0
  Sum : Sum  Inputs=|+-
  pi : Subsystem  mask{kp=kp_align, ki=ki_align, lim_up=lim_up_align, lim_down=lim_down_align}
      mask prompts: ki "ki*ts"
      mask Display:
      | disp('pi()');
      | port_label('input', 1, 'u_ref');
      | port_label('input', 2, 'u');
      | port_label('output', 1, 'y');
  dp : Outport
  wires:
  master_time/1 -> Sum/1
  Constant/1 -> pi/1(u_ref)
  local_time/1 -> Sum/2
  Sum/1 -> pi/2(u)
  pi/1(y) -> dp/1

== system two_time_domains/pwm_alignment_ctrl/phase_compensation_4/alignment_pictrl ==
  local_time : Inport
  master_time : Inport  Port=2
  Constant : Constant  Value=0
  Sum : Sum  Inputs=|+-
  pi : Subsystem  mask{kp=kp_align, ki=ki_align, lim_up=lim_up_align, lim_down=lim_down_align}
      mask prompts: ki "ki*ts"
      mask Display:
      | disp('pi()');
      | port_label('input', 1, 'u_ref');
      | port_label('input', 2, 'u');
      | port_label('output', 1, 'y');
  dp : Outport
  wires:
  master_time/1 -> Sum/1
  Constant/1 -> pi/1(u_ref)
  local_time/1 -> Sum/2
  Sum/1 -> pi/2(u)
  pi/1(y) -> dp/1

== system two_time_domains/pwm_alignment_ctrl/phase_compensation_1/alignment_pictrl/pi ==
  u_ref : Inport
  u : Inport  Port=2
  1/Ti : Gain  Gain=kp  SaturateOnIntegerOverflow=on  OutDataTypeStr=Inherit: Same as input  ParamDataTypeStr=Inherit: Same as input
  Saturation : Saturate  UpperLimit=lim_up  LowerLimit=lim_down
  Sum1 : Sum  Inputs=+++  SaturateOnIntegerOverflow=on
  Sum2 : Sum  Inputs=-+  SaturateOnIntegerOverflow=on
  Sum3 : Sum  Inputs=-+  SaturateOnIntegerOverflow=on
  Unit Delay4 : UnitDelay  SampleTime=-1  HasFrameUpgradeWarning=on
  kp : Gain  Gain=ki  SaturateOnIntegerOverflow=on  OutDataTypeStr=Inherit: Same as input  ParamDataTypeStr=Inherit: Same as input
  y : Outport
  wires:
  1/Ti/1 -> Sum1/1, Sum3/1
  kp/1 -> Sum1/2
  Sum3/1 -> Unit Delay4/1
  Unit Delay4/1 -> Sum1/3
  u_ref/1 -> Sum2/2
  u/1 -> Sum2/1
  Sum2/1 -> kp/1, 1/Ti/1
  Sum1/1 -> Saturation/1
  Saturation/1 -> Sum3/2, y/1

== system two_time_domains/pwm_alignment_ctrl/phase_compensation_2/alignment_pictrl/pi ==
  u_ref : Inport
  u : Inport  Port=2
  1/Ti : Gain  Gain=kp  SaturateOnIntegerOverflow=on  OutDataTypeStr=Inherit: Same as input  ParamDataTypeStr=Inherit: Same as input
  Saturation : Saturate  UpperLimit=lim_up  LowerLimit=lim_down
  Sum1 : Sum  Inputs=+++  SaturateOnIntegerOverflow=on
  Sum2 : Sum  Inputs=-+  SaturateOnIntegerOverflow=on
  Sum3 : Sum  Inputs=-+  SaturateOnIntegerOverflow=on
  Unit Delay4 : UnitDelay  SampleTime=-1  HasFrameUpgradeWarning=on
  kp : Gain  Gain=ki  SaturateOnIntegerOverflow=on  OutDataTypeStr=Inherit: Same as input  ParamDataTypeStr=Inherit: Same as input
  y : Outport
  wires:
  1/Ti/1 -> Sum1/1, Sum3/1
  kp/1 -> Sum1/2
  Sum3/1 -> Unit Delay4/1
  Unit Delay4/1 -> Sum1/3
  u_ref/1 -> Sum2/2
  u/1 -> Sum2/1
  Sum2/1 -> kp/1, 1/Ti/1
  Sum1/1 -> Saturation/1
  Saturation/1 -> Sum3/2, y/1

== system two_time_domains/pwm_alignment_ctrl/phase_compensation_3/alignment_pictrl/pi ==
  u_ref : Inport
  u : Inport  Port=2
  1/Ti : Gain  Gain=kp  SaturateOnIntegerOverflow=on  OutDataTypeStr=Inherit: Same as input  ParamDataTypeStr=Inherit: Same as input
  Saturation : Saturate  UpperLimit=lim_up  LowerLimit=lim_down
  Sum1 : Sum  Inputs=+++  SaturateOnIntegerOverflow=on
  Sum2 : Sum  Inputs=-+  SaturateOnIntegerOverflow=on
  Sum3 : Sum  Inputs=-+  SaturateOnIntegerOverflow=on
  Unit Delay4 : UnitDelay  SampleTime=-1  HasFrameUpgradeWarning=on
  kp : Gain  Gain=ki  SaturateOnIntegerOverflow=on  OutDataTypeStr=Inherit: Same as input  ParamDataTypeStr=Inherit: Same as input
  y : Outport
  wires:
  1/Ti/1 -> Sum1/1, Sum3/1
  kp/1 -> Sum1/2
  Sum3/1 -> Unit Delay4/1
  Unit Delay4/1 -> Sum1/3
  u_ref/1 -> Sum2/2
  u/1 -> Sum2/1
  Sum2/1 -> kp/1, 1/Ti/1
  Sum1/1 -> Saturation/1
  Saturation/1 -> Sum3/2, y/1

== system two_time_domains/pwm_alignment_ctrl/phase_compensation_4/alignment_pictrl/pi ==
  u_ref : Inport
  u : Inport  Port=2
  1/Ti : Gain  Gain=kp  SaturateOnIntegerOverflow=on  OutDataTypeStr=Inherit: Same as input  ParamDataTypeStr=Inherit: Same as input
  Saturation : Saturate  UpperLimit=lim_up  LowerLimit=lim_down
  Sum1 : Sum  Inputs=+++  SaturateOnIntegerOverflow=on
  Sum2 : Sum  Inputs=-+  SaturateOnIntegerOverflow=on
  Sum3 : Sum  Inputs=-+  SaturateOnIntegerOverflow=on
  Unit Delay4 : UnitDelay  SampleTime=-1  HasFrameUpgradeWarning=on
  kp : Gain  Gain=ki  SaturateOnIntegerOverflow=on  OutDataTypeStr=Inherit: Same as input  ParamDataTypeStr=Inherit: Same as input
  y : Outport
  wires:
  1/Ti/1 -> Sum1/1, Sum3/1
  kp/1 -> Sum1/2
  Sum3/1 -> Unit Delay4/1
  Unit Delay4/1 -> Sum1/3
  u_ref/1 -> Sum2/2
  u/1 -> Sum2/1
  Sum2/1 -> kp/1, 1/Ti/1
  Sum1/1 -> Saturation/1
  Saturation/1 -> Sum3/2, y/1

== matlab function two_time_domains/pwm domains/PWM generator_AFE2/MATLAB Function ==
  data: t input; y output; phase input; period input
function y = ramp_up_down(t,phase,period)
x = sin(2*pi/period*t - phase -pi/2);
y = asin(x)/pi + 1/2;

== matlab function two_time_domains/pwm domains/PWM generator_AFE2/MATLAB Function1 ==
  data: sampling_time input; period input; ramp_up_down input; trgo output
function trgo = trgo_gen(sampling_time, period, ramp_up_down)

if period <= 20e-6
    period = 20e-6;
end
th = sampling_time/period*2;

if (((ramp_up_down >= 0) && (ramp_up_down <= th)) || ...
        ((ramp_up_down <= 1) && (ramp_up_down >= 1-th)))
    trgo = 1;
else
    trgo = 0;
end

== matlab function two_time_domains/pwm domains/PWM generator_INV1/MATLAB Function ==
  data: t input; y output; phase input; period input
function y = ramp_up_down(t,phase,period)
x = sin(2*pi/period*t - phase -pi/2);
y = asin(x)/pi + 1/2;

== matlab function two_time_domains/pwm domains/PWM generator_INV1/MATLAB Function1 ==
  data: sampling_time input; period input; ramp_up_down input; trgo output
function trgo = trgo_gen(sampling_time, period, ramp_up_down)

if period <= 20e-6
    period = 20e-6;
end
th = sampling_time/period*2;

if (((ramp_up_down >= 0) && (ramp_up_down <= th)) || ...
        ((ramp_up_down <= 1) && (ramp_up_down >= 1-th)))
    trgo = 1;
else
    trgo = 0;
end

== matlab function two_time_domains/pwm domains/PWM generator_INV2/MATLAB Function ==
  data: t input; y output; phase input; period input
function y = ramp_up_down(t,phase,period)
x = sin(2*pi/period*t - phase -pi/2);
y = asin(x)/pi + 1/2;

== matlab function two_time_domains/pwm domains/PWM generator_INV2/MATLAB Function1 ==
  data: sampling_time input; period input; ramp_up_down input; trgo output
function trgo = trgo_gen(sampling_time, period, ramp_up_down)

if period <= 20e-6
    period = 20e-6;
end
th = sampling_time/period*2;

if (((ramp_up_down >= 0) && (ramp_up_down <= th)) || ...
        ((ramp_up_down <= 1) && (ramp_up_down >= 1-th)))
    trgo = 1;
else
    trgo = 0;
end

== matlab function two_time_domains/pwm domains/PWM generator_AFE1/MATLAB Function ==
  data: t input; y output; phase input; period input
function y = ramp_up_down(t,phase,period)
x = sin(2*pi/period*t - phase -pi/2);
y = asin(x)/pi + 1/2;

== matlab function two_time_domains/pwm domains/PWM generator_AFE1/MATLAB Function1 ==
  data: sampling_time input; period input; ramp_up_down input; trgo output
function trgo = trgo_gen(sampling_time, period, ramp_up_down)

if period <= 20e-6
    period = 20e-6;
end
th = sampling_time/period*2;

if (((ramp_up_down >= 0) && (ramp_up_down <= th)) || ...
        ((ramp_up_down <= 1) && (ramp_up_down >= 1-th)))
    trgo = 1;
else
    trgo = 0;
end
